simulink model "Se_Block"  (R2017b)
settings: Solver=FixedStepAuto  StartTime=0.0  StopTime=inf  RelTol=1e-3
libraries: realtime_pacer_lib x1
settings Model: Creator=hattanbadyah  LastModifiedBy=hattanbadyah
settings CodeAppCC: StateflowObjectComments=on

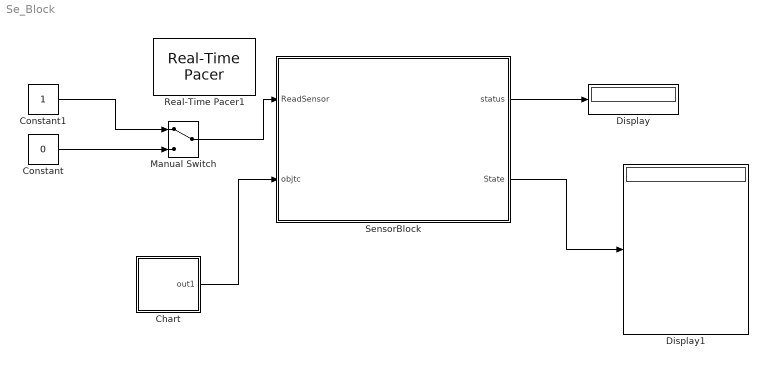
== system Se_Block ==
  Chart : Stateflow chart  TreatAsAtomicUnit=on
  Constant : Constant  Value=0
  Constant1 : Constant
  Display : Display
  Display1 : Display
  Manual Switch : ManualSwitch
  Real-Time Pacer1 : realtime_pacer_lib/Real-Time Pacer  simTimePerRealTime=1
  SensorBlock : Stateflow chart  TreatAsAtomicUnit=on
  wires:
  Manual Switch/1 -> SensorBlock/1(ReadSensor)
  Constant/1 -> Manual Switch/2
  Constant1/1 -> Manual Switch/1
  SensorBlock/1(status) -> Display/1
  SensorBlock/2(State) -> Display1/1
  Chart/1(out1) -> SensorBlock/2(objtc)

== stateflow chart Se_Block/SensorBlock ==
  state A
  state Start
    entry, during:
    coder.extrinsic('evalin')
    so=evalin('base','objWs');
    status = 0
  state Sensor
    entry, during:
    coder.extrinsic('RangeStateRoomba');
    State=RangeStateRoomba(so);
    status = 1;
  (default) -> A
  A -> Start : [objtc==1]
  Start -> Sensor : [ReadSensor==1]
  Sensor -> Start : [ReadSensor==0]
  data: ReadSensor input; status output; so local; State output double size=6; objtc input

== stateflow chart Se_Block/Chart ==
  state A
    en,du:
    tcpInit;
    out1 = 1;
  (default) -> A
  data: out1 output
  function tcpInit:
    | function tcpInit
    | coder.extrinsic('tcpip');
    | coder.extrinsic('assignin');
    | persistent obj
    | if isempty(obj)
    |     obj=tcpip('10.0.0.1',9001);
    |     set(obj,'Terminator','LF')
    |     set(obj,'InputBufferSize',1000)
    |     set(obj, 'Timeout', .5)
    |     set(obj, 'ByteOrder','bigEndian');
    |     assignin('base','objWs',obj);
    |     
    | fopen(obj);
    |     % Start!
    | Start=[128];
    | fwrite(obj,Start);
    | pause(.1)
    | Mode=[132]
    | fwrite(obj,Mode);
    | pause(.1)
    | 
    | % %Print 'go' on display
    | fwrite(obj, [164, 71, 79, 32, 32]);
    | % make a sound
    | fwrite(obj, [140 1 3 60 20 72 20 84 40 ]); %RoombaInit Song
    | fwrite(obj, [140 2 1 60 20]); % BeepRoomba song
    | fwrite(obj, [140 3 3 84 20 72 30 60 40]); % PowerOffRoomba song
    | fwrite(obj, [141 1]); % play RoombaInit song
    | disp('Robot should display go on 7 segment LED panel and play song.')
    | pause(1);
    | end
